simulink model "pid_final"  (R2020b)
settings: Solver=FixedStepDiscrete  StartTime=0.0  StopTime=Inf  FixedStep=0.001  RelTol=1e-3  EnableMultiTasking=on
libraries: arduinolib x2, simulink x2, pid_lib x1
settings Model: SILPILModeSetting=veronly  ExtModeTrigDuration=2  Creator=aleca  LastModifiedBy=aleca
settings OptimizationCC: EnhancedBackFolding=on  PassReuseOutputArgsAs=Individual arguments  ZeroExternalMemoryAtStartup=off  ZeroInternalMemoryAtStartup=off  MaxStackSize=64  OptimizeBlockOrder=speed  DifferentSizesBufferReuse=on  OptimizationCustomize=off  EfficientTunableParamExpr=on
settings DebuggingCC: ParameterTunabilityLossMsg=error
settings HardwareCC: ProdBitPerInt=16  ProdBitPerPointer=16  ProdBitPerSizeT=16  ProdBitPerPtrDiffT=16  ProdLargestAtomicFloat=None  ProdWordSize=8  ProdHWDeviceType=Atmel->AVR  UseEmbeddedCoderFeatures=off  UseSimulinkCoderFeatures=off
settings SFSimCC: MATLABDynamicMemAlloc=off
settings RTWCC: Description=Embedded Coder  SystemTargetFile=ert.tlc  HardwareBoard=Arduino Mega 2560  TemplateMakefile=ert_default_tmf  Toolchain=Arduino AVR  BuildConfiguration=Faster Runs
settings CodeAppCC: ForceParamTrailComments=on  IgnoreCustomStorageClasses=off  OperatorAnnotations=on  SimulinkDataObjDesc=on  SFDataObjDesc=on  InsertBlockDesc=on
settings ERTTargetCC: SupportContinuousTime=on  SupportNonInlinedSFcns=on  SupportVariableSizeSignals=on  ExtModeStaticAllocSize=2048

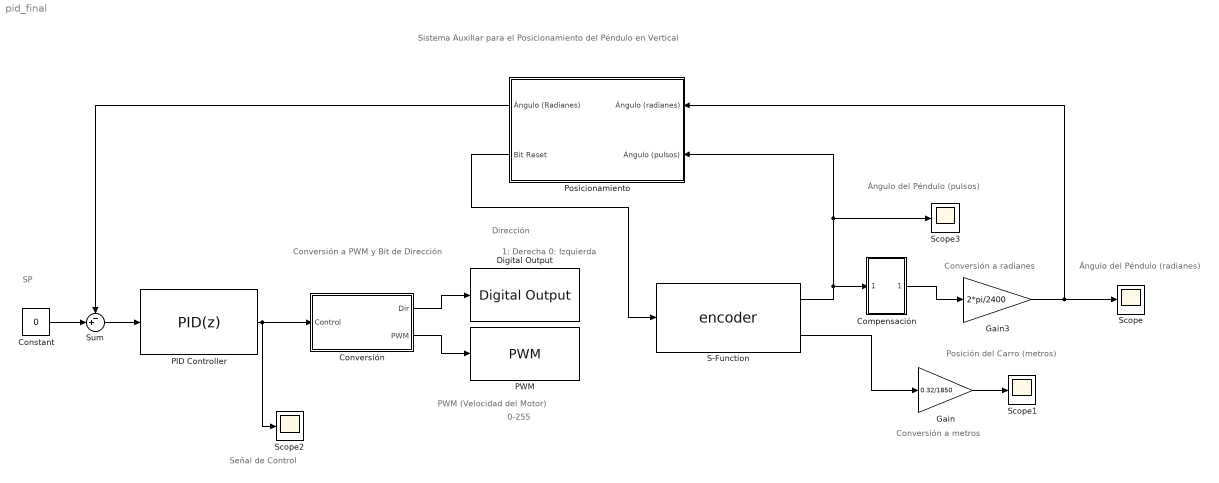
== system pid_final ==
  note: Conversión a PWM y
      | Bit de Dirección
  note: Señal de Control
  note: SP
  note: Sistema Auxiliar para el Posicionamiento del Péndulo en Vertical
  note: Ángulo del Péndulo (radianes)
  note: Posición del Carro (metros)
  note: 0-255
  note: PWM (Velocidad del Motor)
  note: 1: Derecha
      | 0: Izquierda
  note: Dirección
  note: Conversión a metros
  note: Ángulo del Péndulo (pulsos)
  note: Conversión a radianes
  Compensación : Subsystem
  Constant : Constant  Value=0  SampleTime=0.001
  Conversión : Subsystem
  Digital Output : arduinolib/Digital Output  pinNumber=10  Direction=output  blockPlatform=arduino
  Gain : Gain  Gain=0.32/1850
  Gain3 : Gain  Gain=2*pi/2400
  PID Controller : pid_lib/PID Controller  Controller=PID  Form=Parallel  TimeDomain=Discrete-time  UseExternalTs=off  SampleTime=-1  IntegratorMethod=Forward Euler  FilterMethod=Forward Euler  ControllerParametersSource=internal  P=-571  I=-9030  D=-8.7  UseFilter=on  N=925.93  TunerSelectOption=Transfer Function Based (PID Tuner App)  InitialConditionSource=internal  InitialConditionForIntegrator=0  InitialConditionForFilter=0  DifferentiatorICPrevScaledInput=0  ExternalReset=none  TrackingMode=off  Kt=1  LimitOutput=off  SatLimitsSource=internal  UpperSaturationLimit=inf  LowerSaturationLimit=-inf  LinearizeAsGain=on  AntiWindupMode=none  Kb=1  POutMin=[]  POutMax=[]  IOutMin=[]  IOutMax=[]  DOutMin=[]  DOutMax=[]  NOutMin=[]  NOutMax=[]  SumOutMin=[]  SumOutMax=[]  SaturationOutMin=[]  SaturationOutMax=[]  PParamMin=[]  PParamMax=[]  IParamMin=[]  IParamMax=[]  DParamMin=[]  DParamMax=[]  NParamMin=[]  NParamMax=[]  KbParamMin=[]  KbParamMax=[]  KtParamMin=[]  KtParamMax=[]  KbOutMin=[]  KbOutMax=[]  KtOutMin=[]  KtOutMax=[]  IntegratorOutMin=[]  IntegratorOutMax=[]  FilterOutMin=[]  FilterOutMax=[]  SumI1OutMin=[]  SumI1OutMax=[]  SumI2OutMin=[]  SumI2OutMax=[]  SumI3OutMin=[]  SumI3OutMax=[]  SumI4OutMin=[]  SumI4OutMax=[]  SumDOutMin=[]  SumDOutMax=[]  DifferentiatorOutMin=[]  DifferentiatorOutMax=[]  FilterDiffOutCoefMin=[]  FilterDiffOutCoefMax=[]  ReciprocalOutMin=[]  ReciprocalOutMax=[]  SumDenOutMin=[]  SumDenOutMax=[]  SumNumOutMin=[]  SumNumOutMax=[]  DivideOutMin=[]  DivideOutMax=[]  UdiffTsProdOutMin=[]  UdiffTsProdOutMax=[]  NTsProdOutMin=[]  NTsProdOutMax=[]  UintegralTsProdOutMin=[]  UintegralTsProdOutMax=[]  UngainTsProdOutMin=[]  UngainTsProdOutMax=[]  IntegratorContinuousStateAttributes=''  IntegratorStateMustResolveToSignalObject=off  IntegratorRTWStateStorageClass=Auto  FilterContinuousStateAttributes=''  FilterStateMustResolveToSignalObject=off  FilterRTWStateStorageClass=Auto  ParallelPVariant=InternalParameters  IdealPVariant=Disabled  IVariant=InternalParameters  DVariant=InternalParameters  IntegratorVariant=Discrete  SatVariant=Disabled  AWVariant=Passthrough  PCopyVariant=Disabled  TRVariant=Disabled  FdbkBlocksVariant=Forward  IdealPFdbkVariant=Disabled  SatFdbkVariant=Disabled  DerivativeFilterVariant=ForwardEulerFilter  NVariant=InternalParameters  NCopyVariant=Disabled  FilterICVariant=InternalICsFilter  IntegratorICVariant=InternalICs  ExternalResetVariant=Disabled  TRSumVariant=Passthrough  SumFdbkVariant=Disabled  SumVariant=Sum_PID  TsampFilterVariant=InternalTs  TsampNgainVariant=Passthrough  TsampIntegralVariant=Passthrough  ExternalSaturationOutDataTypeStr=Inherit: Same as second input
  PWM : arduinolib/PWM  pinNumber=9  frequencyType=Default  desiredFrequency=490.2  achievableFrequency=490.2
  Posicionamiento : Subsystem
  S-Function : S-Function  FunctionName=encoder  SFunctionModules='encoder_wrapper'  SFunctionDeploymentMode=off  EnableBusSupport=off
  Scope{,1..3} (4 alike) : Scope
  Sum : Sum  Inputs=-+|
  wires:
  Gain/1 -> Scope1/1
  S-Function/2 -> Gain/1
  PID Controller/1 -> Conversión/1(Control), Scope2/1
  Sum/1 -> PID Controller/1
  Constant/1 -> Sum/2
  Gain3/1 -> Posicionamiento/1(Ángulo (radianes)), Scope/1
  S-Function/1 -> Compensación/1(In1), Posicionamiento/2(Ángulo (pulsos)), Scope3/1
  Posicionamiento/1(Ángulo (Radianes)) -> Sum/1
  Posicionamiento/2(Bit Reset) -> S-Function/1
  Conversión/1(Dir) -> Digital Output/1
  Conversión/2(PWM) -> PWM/1
  Compensación/1(Out1) -> Gain3/1

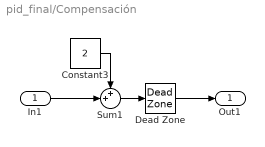
== system pid_final/Compensación ==
  In1 : Inport
  Constant3 : Constant  Value=2  SampleTime=-1
  Dead Zone : DeadZone  LowerValue=-1  UpperValue=1  SaturateOnIntegerOverflow=on
  Sum1 : Sum  Inputs=++|
  Out1 : Outport
  wires:
  Sum1/1 -> Dead Zone/1
  Constant3/1 -> Sum1/1
  In1/1 -> Sum1/2
  Dead Zone/1 -> Out1/1

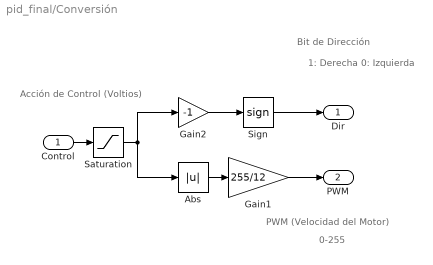
== system pid_final/Conversión ==
  note: Acción de Control
      | (Voltios)
  note: Bit de Dirección
  note: 1: Derecha
      | 0: Izquierda
  note: 0-255
  note: PWM (Velocidad del Motor)
  Control : Inport
  Abs : Abs
  Gain1 : Gain  Gain=255/12
  Gain2 : Gain  Gain=-1
  Saturation : Saturate  UpperLimit=12  LowerLimit=-12
  Sign : Signum
  Dir : Outport
  PWM : Outport  Port=2
  wires:
  Abs/1 -> Gain1/1
  Gain1/1 -> PWM/1
  Control/1 -> Saturation/1
  Saturation/1 -> Gain2/1, Abs/1
  Sign/1 -> Dir/1
  Gain2/1 -> Sign/1

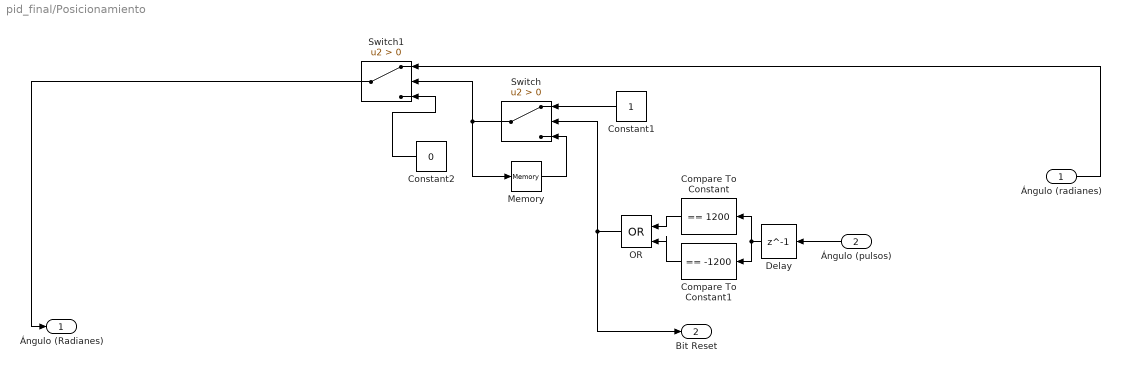
== system pid_final/Posicionamiento ==
  Ángulo (radianes) : Inport
  Ángulo (pulsos) : Inport  Port=2
  Compare To Constant : simulink/Logic and Bit Operations/Compare To Constant  relop===  const=1200  OutDataTypeStr=boolean
  Compare To Constant1 : simulink/Logic and Bit Operations/Compare To Constant  relop===  const=-1200  OutDataTypeStr=boolean
  Constant1 : Constant  OutDataTypeStr=boolean  SampleTime=-1
  Constant2 : Constant  Value=0  SampleTime=-1
  Delay : Delay  DelayLength=1
  Memory : Memory  InheritSampleTime=on
  OR : Logic  Operator=OR  IconShape=distinctive  AllPortsSameDT=off  OutDataTypeStr=boolean
  Switch : Switch  Criteria=u2 > Threshold
  Switch1 : Switch  Criteria=u2 > Threshold
  Ángulo (Radianes) : Outport
  Bit Reset : Outport  Port=2
  wires:
  Memory/1 -> Switch/3
  Switch/1 -> Switch1/2, Memory/1
  Compare To Constant1/1 -> OR/2
  Compare To Constant/1 -> OR/1
  Delay/1 -> Compare To Constant/1, Compare To Constant1/1
  Constant2/1 -> Switch1/3
  OR/1 -> Bit Reset/1, Switch/2
  Ángulo (radianes)/1 -> Switch1/1
  Constant1/1 -> Switch/1
  Switch1/1 -> Ángulo (Radianes)/1
  Ángulo (pulsos)/1 -> Delay/1
